simulink model "FC_IMU_FaultModel"  (R2026a)
settings: Solver=FixedStepAuto  StopTime=15  EnableMultiTasking=on
settings Model: Creator=aylin.edgu  LastModifiedBy=aylin.edgu
settings DebuggingCC: InheritedTsInSrcMsg=none

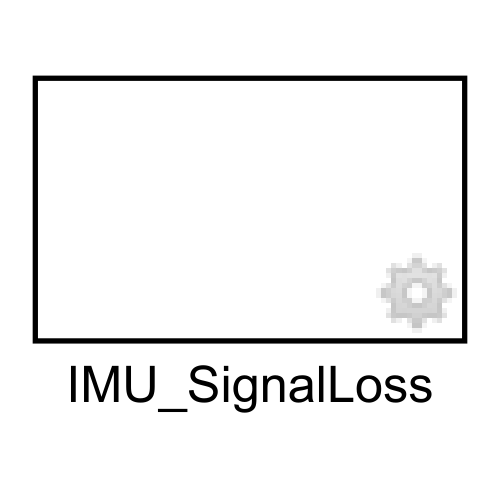
[thumbnail: Simulink's stored preview of the top-level diagram]
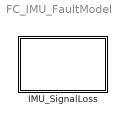
== system FC_IMU_FaultModel ==
  IMU_SignalLoss : Subsystem  TreatAsAtomicUnit=on  IsInjectorSS=on

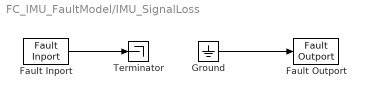
== system FC_IMU_FaultModel/IMU_SignalLoss ==
  Fault Inport : FaultInport
  Fault Outport : FaultOutport
  Ground : Ground
  Terminator : Terminator
  wires:
  Ground/1 -> Fault Outport/1
  Fault Inport/1 -> Terminator/1
